simulink model "SpeedControl"  (R2013b)
settings: Solver=FixedStepDiscrete  SolverMode=SingleTasking  StartTime=0.0  StopTime=inf  FixedStep=0.002  RelTol=1e-3
undefined symbols (not defined in the file): DiscIntNeverNeededParam
libraries: arduinolib x6, simulink x3
settings Model: SimulationMode=external  ExtModeTrigDuration=2  Creator=gcampa  LastModifiedBy=Joshua
settings DataIOCC: SignalLoggingSaveFormat=ModelDataLogs  SaveOutput=off  SaveTime=off
settings OptimizationCC: ExpressionDepthLimit=2147483647  OptimizeModelRefInitCode=on  LifeSpan=1
settings DebuggingCC: SolverPrmCheckMsg=none  MultiTaskDSMMsg=warning  MultiTaskCondExecSysMsg=none  FcnCallInpInsideContextMsg=EnableAllAsWarning  StateNameClashWarn=warning  StrictBusMsg=None
settings HardwareCC: ProdBitPerInt=16  ProdBitPerPointer=16  ProdIntDivRoundTo=Zero  ProdEndianess=LittleEndian  ProdWordSize=8  ProdHWDeviceType=Atmel->AVR
settings RTWCC: SystemTargetFile=realtime.tlc  GenerateMakefile=off  TemplateMakefile=realtime.tmf  Description=Real-Time Toolbox  RTWVerbose=off  ProcessScript=realtime_make_rtw_hook  IncludeERTFirstTime=on
settings CodeAppCC: CustomSymbolStrType=$N$R$M  InternalIdentifier=Classic
settings STFCustomTargetCC: TargetLibSuffix=.a  CodeReplacementLibrary=None  GenerateSampleERTMain=on  ERTCustomFileBanners=on  SupportNonInlinedSFcns=off  SupportVariableSizeSignals=on  MATLABClassNameForMDSCustomization=Simulink.SoftwareTarget.ERTCustomization  GRTInterface=off  SystemTargetFile=realtime.tlc
settings ERTTargetCC: GenerateSampleERTMain=on  ParMdlRefBuildCompliant=off  CompOptLevelCompliant=off  ConcurrentExecutionCompliant=off  CombineOutputUpdateFcns=off  ERTFirstTimeCompliant=off  SupportContinuousTime=on  SupportVariableSizeSignals=on  ModelStepFunctionPrototypeControlCompliant=off  CPPClassGenCompliant=off  ExtModeTransport=3  ExtModeMexFile=ext_serial_win32_comm  ExtModeMexArgs=0 1 9600  InlinedParameterPlacement=NonHierarchical  ERTSrcFileBannerTemplate=realtime_code_template.cgt  ERTHdrFileBannerTemplate=realtime_code_template.cgt  ERTDataSrcFileTemplate=realtime_code_template.cgt  ERTDataHdrFileTemplate=realtime_code_template.cgt  ERTCustomFileTemplate=realtime_file_process.tlc

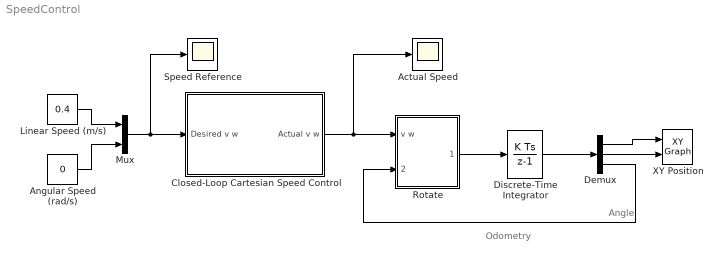
== system SpeedControl ==
  note: Angle
  note: Odometry
  Actual Speed : Scope
      settings: YMin=34.7  YMax=36
  Angular Speed (rad/s) : Constant  Value=0
  Closed-Loop Cartesian Speed Control : Subsystem
  Demux : Demux  Outputs=3
  Discrete-Time Integrator : DiscreteIntegrator  SampleTime=-1  ICPrevOutput=DiscIntNeverNeededParam  ICPrevScaledInput=DiscIntNeverNeededParam
  Linear Speed (m/s) : Constant  Value=0.4
  Mux : Mux  Inputs=2
  Rotate : Subsystem
  Speed Reference : Scope
      settings: YMin=34.7  YMax=36  SaveName=ScopeData2
  XY Position : simulink/Sinks/XY Graph  xmin=-100  xmax=100  ymin=-100  ymax=100  st=-1
  wires:
  Linear Speed (m/s)/1 -> Mux/1
  Rotate/1(vx vy w) -> Discrete-Time Integrator/1
  Demux/1 -> XY Position/1
  Demux/2 -> XY Position/2
  Demux/3 -> Rotate/2(Angle)
  Discrete-Time Integrator/1 -> Demux/1
  Mux/1 -> Speed Reference/1, Closed-Loop Cartesian Speed Control/1(Desired v w)
  Closed-Loop Cartesian Speed Control/1(Actual v w) -> Actual Speed/1, Rotate/1(v w)
  Angular Speed (rad/s)/1 -> Mux/2

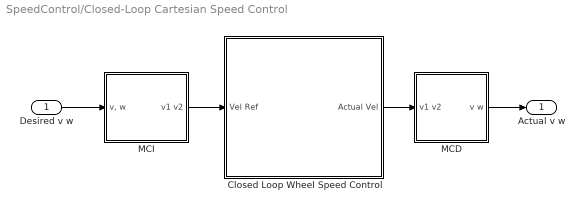
== system SpeedControl/Closed-Loop Cartesian Speed Control ==
  Desired v w : Inport
  Closed Loop Wheel Speed Control : Subsystem
      mask Display: image('imagen_robot.png')
  MCD : Subsystem
  MCI : Subsystem  mask{d=0.22}
      mask prompts: d "Distancia entre ruedas"
  Actual v w : Outport
  wires:
  Closed Loop Wheel Speed Control/1(Actual Vel) -> MCD/1(v1 v2)
  MCD/1(v w) -> Actual v w/1
  MCI/1(v1 v2) -> Closed Loop Wheel Speed Control/1(Vel Ref)
  Desired v w/1 -> MCI/1("v, w")

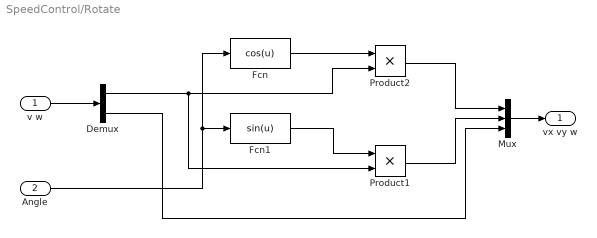
== system SpeedControl/Rotate ==
  v w : Inport
  Angle : Inport  Port=2
  Demux : Demux  Outputs=2
  Fcn : Fcn  Expr=cos(u)
  Fcn1 : Fcn  Expr=sin(u)
  Mux : Mux  Inputs=3
  Product1 : Product
  Product2 : Product
  vx vy w : Outport
  wires:
  Fcn/1 -> Product2/1
  Demux/1 -> Product1/2, Product2/2
  Fcn1/1 -> Product1/1
  Product1/1 -> Mux/2
  Product2/1 -> Mux/1
  Mux/1 -> vx vy w/1
  Demux/2 -> Mux/3
  v w/1 -> Demux/1
  Angle/1 -> Fcn/1, Fcn1/1

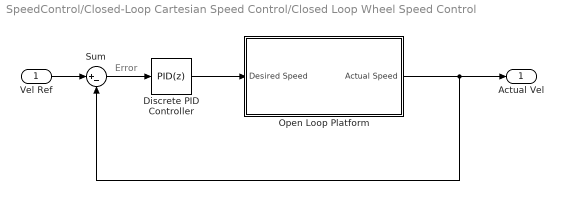
== system SpeedControl/Closed-Loop Cartesian Speed Control/Closed Loop Wheel Speed Control ==
  note: Error
  Vel Ref : Inport
  Discrete PID Controller : simulink/Continuous/PID Controller  Controller=PID  TimeDomain=Discrete-time  SampleTime=-1  IntegratorMethod=Forward Euler  FilterMethod=Forward Euler  Form=Parallel  P=1  I=2  D=0  N=100  InitialConditionSource=internal  InitialConditionForIntegrator=0  InitialConditionForFilter=0  ExternalReset=none  LimitOutput=off  UpperSaturationLimit=inf  LowerSaturationLimit=-inf  LinearizeAsGain=off  AntiWindupMode=none  Kb=1  TrackingMode=off  Kt=1  PParamMin=[]  PParamMax=[]  IParamMin=[]  IParamMax=[]  DParamMin=[]  DParamMax=[]  NParamMin=[]  NParamMax=[]  KbParamMin=[]  KbParamMax=[]  KtParamMin=[]  KtParamMax=[]  POutMin=[]  POutMax=[]  IOutMin=[]  IOutMax=[]  DOutMin=[]  DOutMax=[]  NOutMin=[]  NOutMax=[]  KbOutMin=[]  KbOutMax=[]  KtOutMin=[]  KtOutMax=[]  IntegratorOutMin=[]  IntegratorOutMax=[]  FilterOutMin=[]  FilterOutMax=[]  SumOutMin=[]  SumOutMax=[]  SumI1OutMin=[]  SumI1OutMax=[]  SumI2OutMin=[]  SumI2OutMax=[]  SumI3OutMin=[]  SumI3OutMax=[]  SumDOutMin=[]  SumDOutMax=[]  SaturationOutMin=[]  SaturationOutMax=[]  IntegratorContinuousStateAttributes=''  IntegratorStateMustResolveToSignalObject=off  IntegratorRTWStateStorageClass=Auto  FilterContinuousStateAttributes=''  FilterStateMustResolveToSignalObject=off  FilterRTWStateStorageClass=Auto
  Open Loop Platform : Subsystem
  Sum : Sum  Inputs=|+-
  Actual Vel : Outport
  wires:
  Vel Ref/1 -> Sum/1
  Sum/1 -> Discrete PID Controller/1
  Open Loop Platform/1(Actual Speed) -> Sum/2, Actual Vel/1
  Discrete PID Controller/1 -> Open Loop Platform/1(Desired Speed)

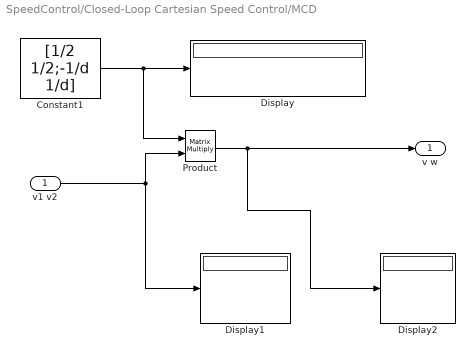
== system SpeedControl/Closed-Loop Cartesian Speed Control/MCD ==
  v1 v2 : Inport
  Constant1 : Constant  Value=[1/2 1/2;-1/d 1/d]  VectorParams1D=off  mask{d=0.22}
      mask prompts: d "distancia"
  Display : Display
  Display1 : Display
  Display2 : Display
  Product : Product  Multiplication=Matrix(*)
  v w : Outport
  wires:
  v1 v2/1 -> Product/2, Display1/1
  Constant1/1 -> Product/1, Display/1
  Product/1 -> v w/1, Display2/1

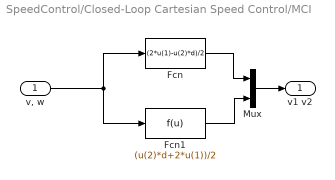
== system SpeedControl/Closed-Loop Cartesian Speed Control/MCI ==
  "v, w" : Inport
  Fcn : Fcn  Expr=(2*u(1)-u(2)*d)/2
  Fcn1 : Fcn  Expr=(u(2)*d+2*u(1))/2
  Mux : Mux  Inputs=2
  v1 v2 : Outport
  wires:
  Fcn/1 -> Mux/1
  Fcn1/1 -> Mux/2
  "v, w"/1 -> Fcn/1, Fcn1/1
  Mux/1 -> v1 v2/1

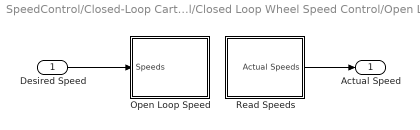
== system SpeedControl/Closed-Loop Cartesian Speed Control/Closed Loop Wheel Speed Control/Open Loop Platform ==
  Desired Speed : Inport
  Open Loop Speed : Subsystem
  Read Speeds : Subsystem
  Actual Speed : Outport
  wires:
  Desired Speed/1 -> Open Loop Speed/1(Speeds)
  Read Speeds/1(Actual Speeds) -> Actual Speed/1

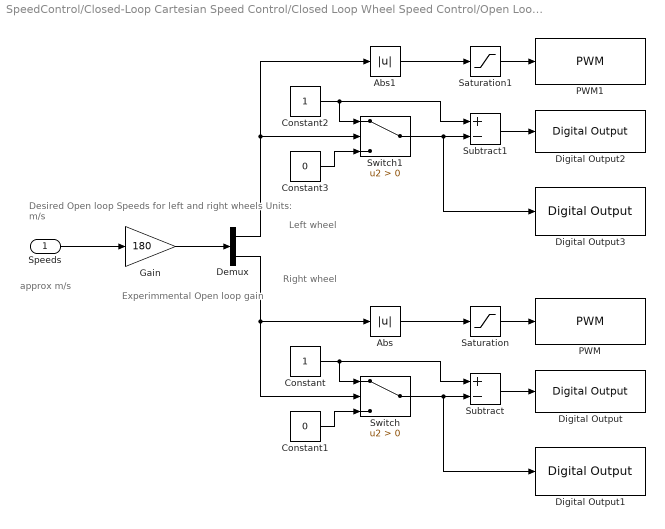
== system SpeedControl/Closed-Loop Cartesian Speed Control/Closed Loop Wheel Speed Control/Open Loop Platform/Open Loop Speed ==
  note: Right wheel
  note: Left wheel
  note: approx m/s
  note: Experimmental
      | Open loop gain
  note: Desired Open loop Speeds for left and right wheels
      | Units: m/s
  Speeds : Inport
  Abs : Abs
  Abs1 : Abs
  Constant : Constant
  Constant1 : Constant  Value=0
  Constant2 : Constant
  Constant3 : Constant  Value=0
  Demux : Demux  Outputs=2
  Digital Output : arduinolib/Digital Output  pinNumber=11
  Digital Output1 : arduinolib/Digital Output  pinNumber=12
  Digital Output2 : arduinolib/Digital Output  pinNumber=9
  Digital Output3 : arduinolib/Digital Output  pinNumber=10
  Gain : Gain  Gain=180
  PWM : arduinolib/PWM  pinNumber=13
  PWM1 : arduinolib/PWM  pinNumber=8
  Saturation : Saturate  UpperLimit=255  LowerLimit=0  OutDataTypeStr=uint8
  Saturation1 : Saturate  UpperLimit=255  LowerLimit=0  OutDataTypeStr=uint8
  Subtract : Sum  Inputs=+-
  Subtract1 : Sum  Inputs=+-
  Switch : Switch  Criteria=u2 > Threshold
  Switch1 : Switch  Criteria=u2 > Threshold
  wires:
  Speeds/1 -> Gain/1
  Abs/1 -> Saturation/1
  Gain/1 -> Demux/1
  Constant/1 -> Subtract/1, Switch/1
  Constant1/1 -> Switch/3
  Switch/1 -> Digital Output1/1, Subtract/2
  Subtract/1 -> Digital Output/1
  Saturation/1 -> PWM/1
  Abs1/1 -> Saturation1/1
  Constant2/1 -> Switch1/1, Subtract1/1
  Constant3/1 -> Switch1/3
  Switch1/1 -> Subtract1/2, Digital Output3/1
  Subtract1/1 -> Digital Output2/1
  Saturation1/1 -> PWM1/1
  Demux/1 -> Abs1/1, Switch1/2
  Demux/2 -> Switch/2, Abs/1

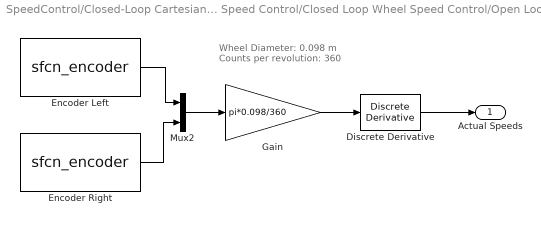
== system SpeedControl/Closed-Loop Cartesian Speed Control/Closed Loop Wheel Speed Control/Open Loop Platform/Read Speeds ==
  note: Wheel Diameter: 0.098 m
      | Counts per revolution: 360
  Discrete Derivative : simulink/Discrete/Discrete Derivative  gainval=1.0  ICPrevScaledInput=0.0  InputProcessing=Inherited  OutMin=[]  OutMax=[]  OutDataType=fixdt(1, 16)  OutScaling=2^-10  DoSatur=off
  Encoder Left : S-Function  InitFcn=try, set_param(gcb,'FunctionName','sfcn_encoder'), end  FunctionName=sfcn_encoder  Parameters=uint8(0),uint8(3),uint8(2)  SFunctionModules=sfcn_encoder_wrapper  EnableBusSupport=off  mask(S-Function Builder){}
      mask init:
      | val = [[.9  0.75 0.75 1 1 .9 .9 1]',[1 1 0.75 0.75 .9 .9 1 .9]'];try , sys = get_param(gcb,'SfunBuilderFcnName');if isempty(sys), sys = get_param(gcb,'FunctionName'); end,catch, sys = get_param(gcb,'FunctionName'); end
      settings: CopyFcn=set_param(gcbh,'LinkStatus','none')  PreSaveFcn=try, set_param(gcb,'FunctionName','sfcn_encoder'), end  OpenFcn=sfunctionwizard(gcbh)
      mask Display: plot(val(:,1),val(:,2)),disp(sys), port_label('output',1,'pos')
  Encoder Right : S-Function  InitFcn=try, set_param(gcb,'FunctionName','sfcn_encoder'), end  FunctionName=sfcn_encoder  Parameters=uint8(1),uint8(19),uint8(18)  SFunctionModules=sfcn_encoder_wrapper  EnableBusSupport=off  mask(S-Function Builder){}
      mask init: same as SpeedControl/Closed-Loop Cartesian Speed Control/Closed Loop Wheel Speed Control/Open Loop Platform/Read Speeds/Encoder Left
      settings: CopyFcn=set_param(gcbh,'LinkStatus','none')  PreSaveFcn=try, set_param(gcb,'FunctionName','sfcn_encoder'), end  OpenFcn=sfunctionwizard(gcbh)
      mask Display: plot(val(:,1),val(:,2)),disp(sys), port_label('output',1,'pos')
  Gain : Gain  Gain=pi*0.098/360  OutDataTypeStr=double
  Mux2 : Mux  Inputs=2
  Actual Speeds : Outport
  wires:
  Gain/1 -> Discrete Derivative/1
  Encoder Left/1 -> Mux2/1
  Encoder Right/1 -> Mux2/2
  Discrete Derivative/1 -> Actual Speeds/1
  Mux2/1 -> Gain/1
